simulink model "modelo_fanplate"  (R2023a)
settings: Solver=VariableStepAuto  StartTime=0.0  StopTime=30  RelTol=1e-3
undefined symbols (not defined in the file): A1, A2, Fg, G1, Jm, Jp, Ka, Kap, Kw, L_m, La, Pos_sat_under, Pos_sat_upper, Ra, V_max, V_min
libraries: simulink x1
settings Model: Creator=hugo  LastModifiedBy=hugo

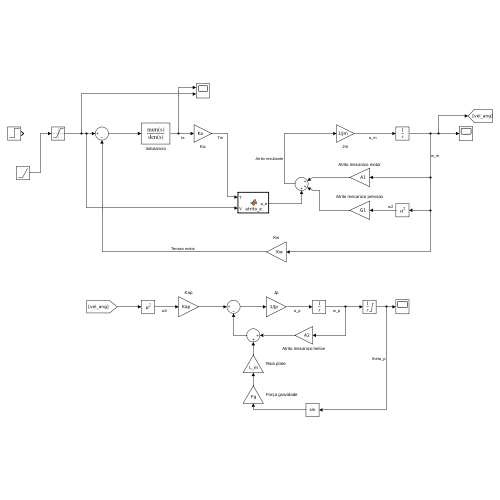
[thumbnail: Simulink's stored preview of the top-level diagram]
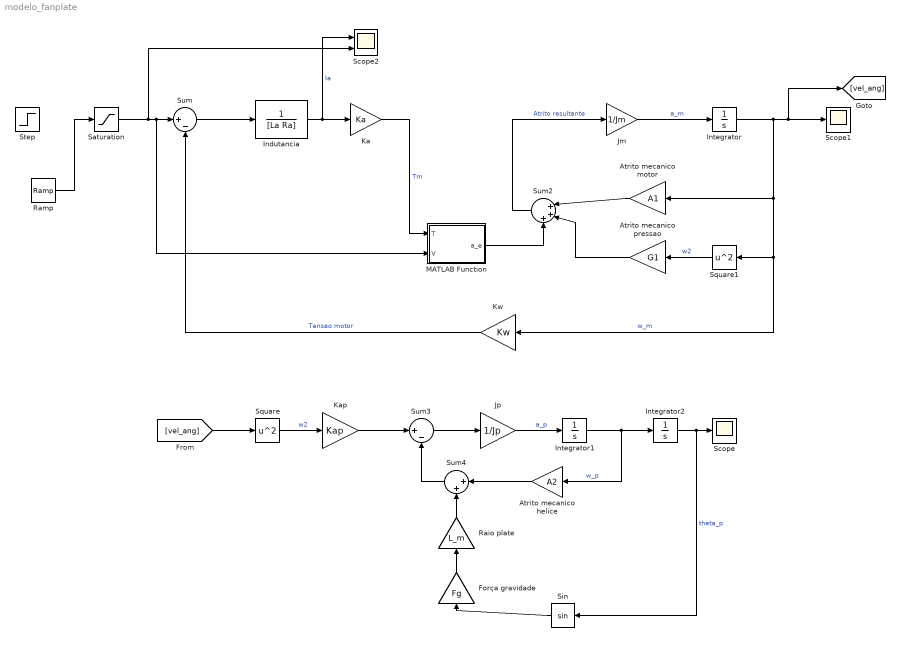
== system modelo_fanplate ==
  Atrito mecanico helice : Gain  Gain=A2
  Atrito mecanico motor : Gain  Gain=A1
  Atrito mecanico pressao : Gain  Gain=G1
  Força gravidade : Gain  Gain=Fg
  Indutancia : TransferFcn  Denominator=[La Ra]
  Integrator : Integrator
  Integrator1 : Integrator
  Integrator2 : Integrator  LimitOutput=on  UpperSaturationLimit=Pos_sat_upper  LowerSaturationLimit=Pos_sat_under
  Jm : Gain  Gain=1/Jm
  Jp : Gain  Gain=1/Jp
  Ka : Gain  Gain=Ka
  Kap : Gain  Gain=Kap
  Kw : Gain  Gain=Kw
  MATLAB Function : MATLAB Function  TreatAsAtomicUnit=on
  Raio plate : Gain  Gain=L_m
  Ramp : simulink/Sources/Ramp  slope=1  start=0  InitialOutput=0
  Saturation : Saturate  UpperLimit=V_max  LowerLimit=V_min
  Scope : Scope
  Scope1 : Scope
  Scope2 : Scope  NumInputPorts=2
  Sin : Trigonometry
  Square : Math  Operator=square
  Square1 : Math  Operator=square
  Step : Step  After=9.1  SampleTime=0
  Sum : Sum  Inputs=|+-
  Sum2 : Sum  Inputs=|+++
  Sum3 : Sum  Inputs=|+-
  Sum4 : Sum  Inputs=|++
  wires:
  Sum/1 -> Indutancia/1
  Indutancia/1 -> Scope2/1, Ka/1  "Ia"
  Ka/1 -> MATLAB Function/1(T)  "Tm"
  Jm/1 -> Integrator/1  "a_m"
  Integrator/1 -> [vel_ang], Scope1/1, Square1/1, Kw/1, Atrito mecanico motor/1  "w_m"
  Kw/1 -> Sum/2  "Tensao motor"
  Square/1 -> Kap/1  "w2"
  Kap/1 -> Sum3/1
  Sum4/1 -> Sum3/2
  Atrito mecanico helice/1 -> Sum4/1
  Raio plate/1 -> Sum4/2
  Sum3/1 -> Jp/1
  Jp/1 -> Integrator1/1  "a_p"
  Integrator1/1 -> Atrito mecanico helice/1, Integrator2/1  "w_p"
  Integrator2/1 -> Sin/1, Scope/1  "theta_p"
  Força gravidade/1 -> Raio plate/1
  Sin/1 -> Força gravidade/1
  Atrito mecanico motor/1 -> Sum2/1
  Atrito mecanico pressao/1 -> Sum2/2
  MATLAB Function/1(a_e) -> Sum2/3
  Square1/1 -> Atrito mecanico pressao/1  "w2"
  Sum2/1 -> Jm/1  "Atrito resultante"
  Saturation/1 -> Scope2/2, MATLAB Function/2(V), Sum/1
  [vel_ang] -> Square/1
  Ramp/1 -> Saturation/1

== matlab function modelo_fanplate/MATLAB Function ==
  data: T input; a_e output; V input
function a_e = atrito_e(T,V)

if V <3
    a_e = 0;
else
    a_e = T;
end

end
